simulink model "PhaseLockedLoop"  (R2025b)
settings: Solver=VariableStepAuto  StartTime=0.0  StopTime=100  RelTol=1e-3
values from neighbouring files (symbols this model uses):
  fo = 1000    [startup.m]
  fref = 500    [startup.m]
  Ki = 80    [startup.m]
  Kp = 800    [startup.m]
  Kpd_scale = 1    [startup.m]
  Kvco = 5e+6    (= 5000000)    [startup.m]
  tau = 1/Wc    (= 0.00176838825658)    [startup.m]
  Wc = 2*pi*fc    (= 565.486677646)    [startup.m]
undefined symbols (not defined in the file or in its folder): C, Icp
libraries: simulink_extras x3, simulink x1
settings Model: PacingRate=100  Creator=Chetan  LastModifiedBy=Chetan

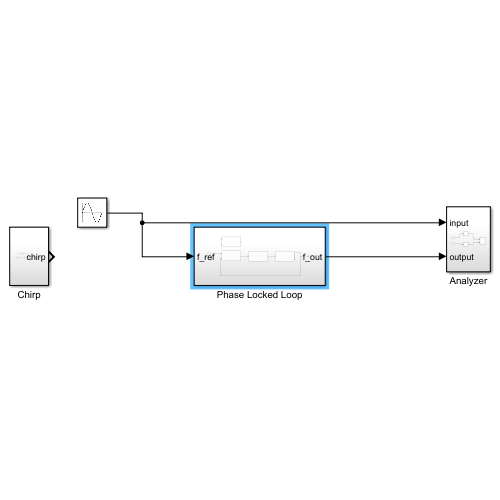
[thumbnail: Simulink's stored preview of the top-level diagram]
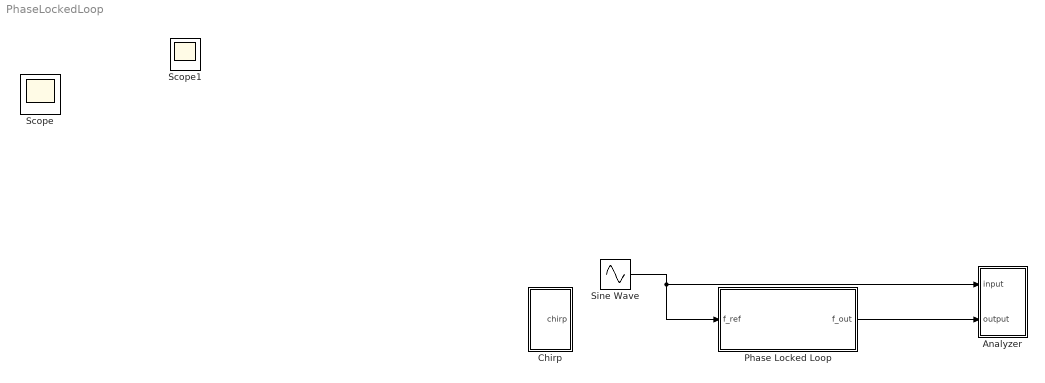
== system PhaseLockedLoop ==
  Analyzer : Subsystem
  Chirp : Subsystem
  Phase Locked Loop : Subsystem
  Sine Wave : Sin  Frequency=2*pi*fref  SampleTime=0  VectorParams1D=off
  Scope : Scope
      settings: ActiveDisplayYMinimum=-6.30574634333698  ActiveDisplayYMaximum=4.9447781799252981
  Scope1 : Scope
      settings: ActiveDisplayYMinimum=-585421.58722594846  ActiveDisplayYMaximum=380292.44329244131
  wires:
  Phase Locked Loop/1(f_out) -> Analyzer/2(output)
  Sine Wave/1 -> Phase Locked Loop/1(f_ref), Analyzer/1(input)

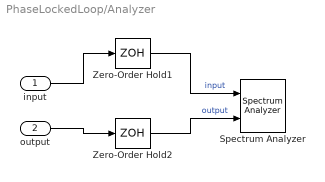
== system PhaseLockedLoop/Analyzer ==
  input : Inport
  output : Inport  Port=2
  Spectrum Analyzer : SpectrumAnalyzer  NumInputPorts=2  WindowPosition=[398.000000,218.000000,1061.000000,702.000000,]  ScopeFrameLocation=window  PlotAsTwoSidedSpectrum=off  WindowInvariantSamplesPerUpdate=on  Span=5  StartFrequency=0  StopFrequency=1000  MaximizeAxes=On  YLimits=[-47.5777 33.442]  ColorLimits=[NaN NaN]  ShowLegend=on  SelectedToolstripTab=spectrumAnalyzerToolstrip.measurementsTab
      settings: OpenAtSimulationStart=off
  Zero-Order Hold1 : ZeroOrderHold  SampleTime=-1
  Zero-Order Hold2 : ZeroOrderHold  SampleTime=-1
  wires:
  Zero-Order Hold1/1 -> Spectrum Analyzer/1  "input"
  output/1 -> Zero-Order Hold2/1
  Zero-Order Hold2/1 -> Spectrum Analyzer/2  "output"
  input/1 -> Zero-Order Hold1/1

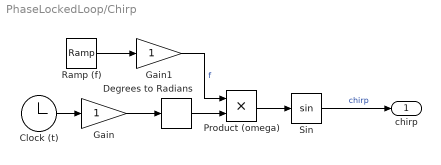
== system PhaseLockedLoop/Chirp ==
  Clock (t) : Clock
  Degrees to Radians : simulink_extras/Transformations/Degrees to Radians
  Gain : Gain
  Gain1 : Gain
  Product (omega) : Product
  Ramp (f) : simulink/Sources/Ramp  slope=1  start=0  InitialOutput=0
  Sin : Trigonometry
  chirp : Outport
  wires:
  Clock (t)/1 -> Gain/1
  Ramp (f)/1 -> Gain1/1
  Sin/1 -> chirp/1  "chirp"
  Product (omega)/1 -> Sin/1
  Degrees to Radians/1 -> Product (omega)/2
  Gain/1 -> Degrees to Radians/1
  Gain1/1 -> Product (omega)/1  "f"

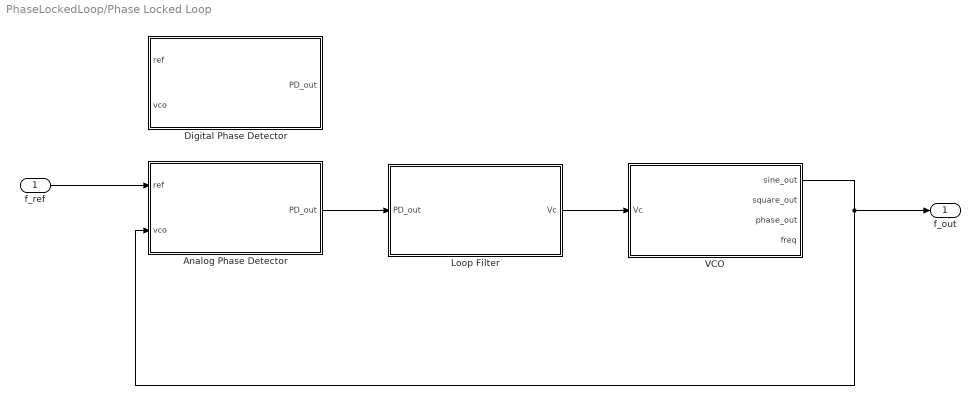
== system PhaseLockedLoop/Phase Locked Loop ==
  f_ref : Inport
  Analog Phase Detector : Subsystem
  Digital Phase Detector : Subsystem
  Loop Filter : Subsystem
  VCO : Subsystem
  f_out : Outport
  wires:
  VCO/1(sine_out) -> Analog Phase Detector/2(vco), f_out/1
  f_ref/1 -> Analog Phase Detector/1(ref)
  Loop Filter/1(Vc) -> VCO/1(Vc)
  Analog Phase Detector/1(PD_out) -> Loop Filter/1(PD_out)

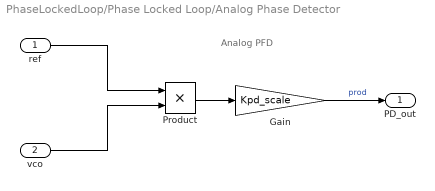
== system PhaseLockedLoop/Phase Locked Loop/Analog Phase Detector ==
  note: Analog PFD
  ref : Inport
  vco : Inport  Port=2
  Gain : Gain  Gain=Kpd_scale
  Product : Product
  PD_out : Outport
  wires:
  ref/1 -> Product/1
  vco/1 -> Product/2
  Product/1 -> Gain/1
  Gain/1 -> PD_out/1  "prod"

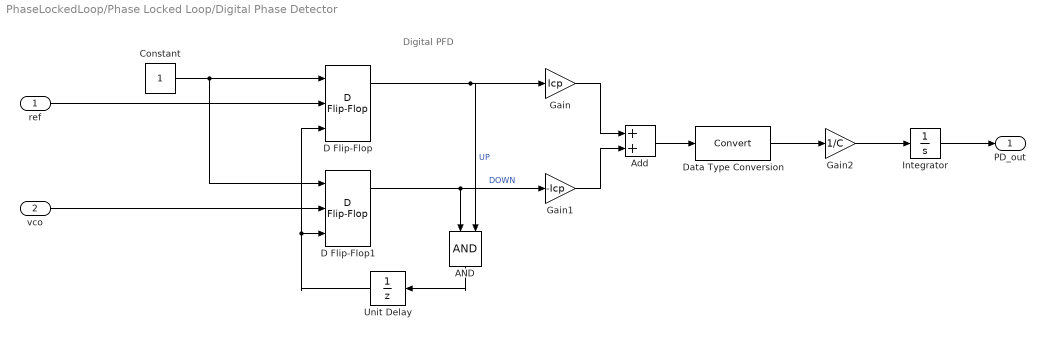
== system PhaseLockedLoop/Phase Locked Loop/Digital Phase Detector ==
  note: Digital PFD
  ref : Inport
  vco : Inport  Port=2
  AND : Logic  IconShape=distinctive  AllPortsSameDT=off  OutDataTypeStr=boolean
  Add : Sum
  Constant : Constant  OutDataTypeStr=boolean
  D Flip-Flop : simulink_extras/Flip Flops/D Flip-Flop
  D Flip-Flop1 : simulink_extras/Flip Flops/D Flip-Flop
  Data Type Conversion : DataTypeConversion  SaturateOnIntegerOverflow=off  RndMeth=Floor
  Gain : Gain  Gain=Icp
  Gain1 : Gain  Gain=-Icp
  Gain2 : Gain  Gain=1/C
  Integrator : Integrator
  Unit Delay : UnitDelay  SampleTime=-1  HasFrameUpgradeWarning=on
  PD_out : Outport
  wires:
  ref/1 -> D Flip-Flop/2
  vco/1 -> D Flip-Flop1/2
  Constant/1 -> D Flip-Flop1/1, D Flip-Flop/1
  D Flip-Flop/1 -> Gain/1, AND/2  "UP"
  D Flip-Flop1/1 -> Gain1/1, AND/1  "DOWN"
  AND/1 -> Unit Delay/1
  Gain/1 -> Add/1
  Gain1/1 -> Add/2
  Add/1 -> Data Type Conversion/1
  Gain2/1 -> Integrator/1
  Integrator/1 -> PD_out/1
  Data Type Conversion/1 -> Gain2/1
  Unit Delay/1 -> D Flip-Flop/3, D Flip-Flop1/3

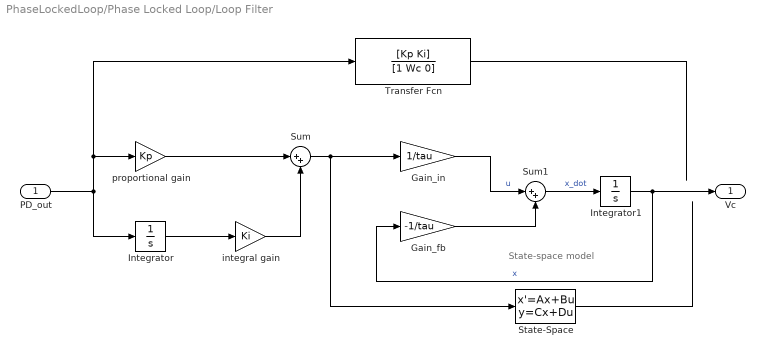
== system PhaseLockedLoop/Phase Locked Loop/Loop Filter ==
  note: State-space model
  PD_out : Inport
  Gain_fb : Gain  Gain=-1/tau
  Gain_in : Gain  Gain=1/tau
  Integrator : Integrator
  Integrator1 : Integrator
  State-Space : StateSpace  A=-1/tau  B=1/tau  D=0  InitialCondition=0
  Sum : Sum  Inputs=|++
  Sum1 : Sum  Inputs=|++
  Transfer Fcn : TransferFcn  Numerator=[Kp Ki]  Denominator=[1 Wc 0]
  integral gain : Gain  Gain=Ki
  proportional gain : Gain  Gain=Kp
  Vc : Outport
  wires:
  PD_out/1 -> Transfer Fcn/1, proportional gain/1, Integrator/1
  Sum/1 -> State-Space/1, Gain_in/1
  Integrator/1 -> integral gain/1
  integral gain/1 -> Sum/2
  proportional gain/1 -> Sum/1
  Gain_in/1 -> Sum1/1  "u"
  Gain_fb/1 -> Sum1/2
  Sum1/1 -> Integrator1/1  "x_dot"
  Transfer Fcn/1 -> ?
  State-Space/1 -> ?
  Integrator1/1 -> Vc/1, Gain_fb/1  "x"

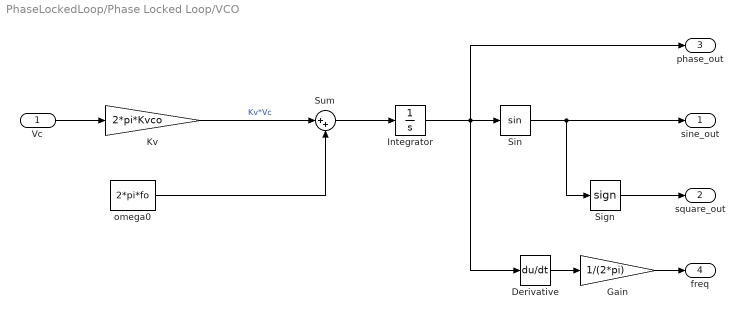
== system PhaseLockedLoop/Phase Locked Loop/VCO ==
  Vc : Inport
  Derivative : Derivative
  Gain : Gain  Gain=1/(2*pi)
  Integrator : Integrator
  Kv : Gain  Gain=2*pi*Kvco
  Sign : Signum
  Sin : Trigonometry  OutputSignalType=real
  Sum : Sum  Inputs=|++
  omega0 : Constant  Value=2*pi*fo
  sine_out : Outport
  square_out : Outport  Port=2
  phase_out : Outport  Port=3
  freq : Outport  Port=4
  wires:
  Vc/1 -> Kv/1
  Kv/1 -> Sum/1  "Kv*Vc"
  Sum/1 -> Integrator/1
  omega0/1 -> Sum/2
  Sin/1 -> sine_out/1, Sign/1
  Sign/1 -> square_out/1
  Derivative/1 -> Gain/1
  Gain/1 -> freq/1
  Integrator/1 -> Sin/1, phase_out/1, Derivative/1
